simulink model "IEEE14_case"  (R2024b)
settings: Solver=FixedStepAuto  StartTime=0  StopTime=2  FixedStep=1e-7  RelTol=1e-3
values from neighbouring files (symbols this model uses):
  GFL_15_Bva = 0.009    [IEEE14_parameters.m]
  GFL_15_C_bus_pu = 7.179419    [IEEE14_parameters.m]
  GFL_15_f0 = 60    [IEEE14_parameters.m]
  GFL_15_I_id = 691.26967    [IEEE14_parameters.m]
  GFL_15_I_iq = 691.26967    [IEEE14_parameters.m]
  GFL_15_I_od = 45.2207    [IEEE14_parameters.m]
  GFL_15_I_oq = 45.2207    [IEEE14_parameters.m]
  GFL_15_I_pll = 0.78    [IEEE14_parameters.m]
  GFL_15_Kdi = 0.09    [IEEE14_parameters.m]
  GFL_15_Kdo = 0.9    [IEEE14_parameters.m]
  GFL_15_Kqi = 0.09    [IEEE14_parameters.m]
  GFL_15_Kqo = 0.9    [IEEE14_parameters.m]
  GFL_15_Lg_pu = 0.631447    [IEEE14_parameters.m]
  GFL_15_mode = 1    [IEEE14_parameters.m]
  GFL_15_P_id = 3.7166    [IEEE14_parameters.m]
  GFL_15_P_iq = 3.7166    [IEEE14_parameters.m]
  GFL_15_P_od = 0.4798    [IEEE14_parameters.m]
  GFL_15_P_oq = 0.4798    [IEEE14_parameters.m]
  GFL_15_P_pll = 290.42    [IEEE14_parameters.m]
  GFL_15_Qe_ref = 0.2    [IEEE14_parameters.m]
  GFL_15_Rg_pu = 0.024016    [IEEE14_parameters.m]
  GFL_15_Sbase = 1.000000e+4    (= 10000)    [IEEE14_parameters.m]
  GFL_15_Tdi = 0.01    [IEEE14_parameters.m]
  GFL_15_Tdo = 0.2    [IEEE14_parameters.m]
  GFL_15_Tqi = 0.01    [IEEE14_parameters.m]
  GFL_15_Tqo = 0.2    [IEEE14_parameters.m]
  GFL_15_Vbase = 380    [IEEE14_parameters.m]
  GFL_15_Vdc_ref = 1.011475    [IEEE14_parameters.m]
  GFL_15_Vdcbase = 700    [IEEE14_parameters.m]
  GFL_15_vq_ref = 0    [IEEE14_parameters.m]
  GFL_16_Bva = 0.002    [IEEE14_parameters.m]
  GFL_16_C_bus_pu = 7.179419    [IEEE14_parameters.m]
  GFL_16_f0 = 60    [IEEE14_parameters.m]
  GFL_16_I_id = 691.26967    [IEEE14_parameters.m]
  GFL_16_I_iq = 691.26967    [IEEE14_parameters.m]
  GFL_16_I_od = 45.2207    [IEEE14_parameters.m]
  GFL_16_I_oq = 45.2207    [IEEE14_parameters.m]
  GFL_16_I_pll = 0.78    [IEEE14_parameters.m]
  GFL_16_Kdi = 0.05    [IEEE14_parameters.m]
  GFL_16_Kdo = 0.5    [IEEE14_parameters.m]
  GFL_16_Kqi = 0.05    [IEEE14_parameters.m]
  GFL_16_Kqo = 0.5    [IEEE14_parameters.m]
  GFL_16_Lg_pu = 0.631447    [IEEE14_parameters.m]
  GFL_16_mode = 1    [IEEE14_parameters.m]
  GFL_16_P_id = 3.7166    [IEEE14_parameters.m]
  GFL_16_P_iq = 3.7166    [IEEE14_parameters.m]
  GFL_16_P_od = 0.4798    [IEEE14_parameters.m]
  GFL_16_P_oq = 0.4798    [IEEE14_parameters.m]
  GFL_16_P_pll = 290.42    [IEEE14_parameters.m]
  GFL_16_Qe_ref = 0.2    [IEEE14_parameters.m]
  GFL_16_Rg_pu = 0.024016    [IEEE14_parameters.m]
  GFL_16_Sbase = 1.000000e+4    (= 10000)    [IEEE14_parameters.m]
  GFL_16_Tdi = 0.01    [IEEE14_parameters.m]
  GFL_16_Tdo = 0.2    [IEEE14_parameters.m]
  GFL_16_Tqi = 0.01    [IEEE14_parameters.m]
  GFL_16_Tqo = 0.2    [IEEE14_parameters.m]
  GFL_16_Vbase = 380    [IEEE14_parameters.m]
  GFL_16_Vdc_ref = 1.01144    [IEEE14_parameters.m]
  GFL_16_Vdcbase = 700    [IEEE14_parameters.m]
  GFL_16_vq_ref = 0    [IEEE14_parameters.m]
  GFL_17_Bva = 0.002    [IEEE14_parameters.m]
  GFL_17_C_bus_pu = 7.179419    [IEEE14_parameters.m]
  GFL_17_f0 = 60    [IEEE14_parameters.m]
  GFL_17_I_id = 691.26967    [IEEE14_parameters.m]
  GFL_17_I_iq = 691.26967    [IEEE14_parameters.m]
  GFL_17_I_od = 45.2207    [IEEE14_parameters.m]
  GFL_17_I_oq = 45.2207    [IEEE14_parameters.m]
  GFL_17_I_pll = 0.78    [IEEE14_parameters.m]
  GFL_17_Kdi = 0.05    [IEEE14_parameters.m]
  GFL_17_Kdo = 0.5    [IEEE14_parameters.m]
  GFL_17_Kqi = 0.05    [IEEE14_parameters.m]
  GFL_17_Kqo = 0.5    [IEEE14_parameters.m]
  GFL_17_Lg_pu = 0.631447    [IEEE14_parameters.m]
  GFL_17_mode = 1    [IEEE14_parameters.m]
  GFL_17_P_id = 3.7166    [IEEE14_parameters.m]
  GFL_17_P_iq = 3.7166    [IEEE14_parameters.m]
  GFL_17_P_od = 0.4798    [IEEE14_parameters.m]
  GFL_17_P_oq = 0.4798    [IEEE14_parameters.m]
  GFL_17_P_pll = 290.42    [IEEE14_parameters.m]
  GFL_17_Qe_ref = 0.2    [IEEE14_parameters.m]
  GFL_17_Rg_pu = 0.024016    [IEEE14_parameters.m]
  GFL_17_Sbase = 1.000000e+4    (= 10000)    [IEEE14_parameters.m]
  GFL_17_Tdi = 0.01    [IEEE14_parameters.m]
  GFL_17_Tdo = 0.2    [IEEE14_parameters.m]
  GFL_17_Tqi = 0.01    [IEEE14_parameters.m]
  GFL_17_Tqo = 0.2    [IEEE14_parameters.m]
  GFL_17_Vbase = 380    [IEEE14_parameters.m]
  GFL_17_Vdc_ref = 1.011632    [IEEE14_parameters.m]
  GFL_17_Vdcbase = 700    [IEEE14_parameters.m]
  GFL_17_vq_ref = 0    [IEEE14_parameters.m]
  GFL_18_Bva = 0.002    [IEEE14_parameters.m]
  GFL_18_C_bus_pu = 7.179419    [IEEE14_parameters.m]
  GFL_18_f0 = 60    [IEEE14_parameters.m]
  GFL_18_I_id = 691.26967    [IEEE14_parameters.m]
  GFL_18_I_iq = 691.26967    [IEEE14_parameters.m]
  GFL_18_I_od = 45.2207    [IEEE14_parameters.m]
  GFL_18_I_oq = 45.2207    [IEEE14_parameters.m]
  GFL_18_I_pll = 0.78    [IEEE14_parameters.m]
  GFL_18_Kdi = 0.05    [IEEE14_parameters.m]
  GFL_18_Kdo = 0.5    [IEEE14_parameters.m]
  GFL_18_Kqi = 0.05    [IEEE14_parameters.m]
  GFL_18_Kqo = 0.5    [IEEE14_parameters.m]
  GFL_18_Lg_pu = 0.631447    [IEEE14_parameters.m]
  GFL_18_mode = 1    [IEEE14_parameters.m]
  GFL_18_P_id = 3.7166    [IEEE14_parameters.m]
  GFL_18_P_iq = 3.7166    [IEEE14_parameters.m]
  GFL_18_P_od = 0.4798    [IEEE14_parameters.m]
  GFL_18_P_oq = 0.4798    [IEEE14_parameters.m]
  GFL_18_P_pll = 290.42    [IEEE14_parameters.m]
  GFL_18_Qe_ref = 0.2    [IEEE14_parameters.m]
  GFL_18_Rg_pu = 0.024016    [IEEE14_parameters.m]
  GFL_18_Sbase = 1.000000e+4    (= 10000)    [IEEE14_parameters.m]
  GFL_18_Tdi = 0.01    [IEEE14_parameters.m]
  GFL_18_Tdo = 0.2    [IEEE14_parameters.m]
  GFL_18_Tqi = 0.01    [IEEE14_parameters.m]
  GFL_18_Tqo = 0.2    [IEEE14_parameters.m]
  GFL_18_Vbase = 380    [IEEE14_parameters.m]
  GFL_18_Vdc_ref = 1.011572    [IEEE14_parameters.m]
  GFL_18_Vdcbase = 700    [IEEE14_parameters.m]
  GFL_18_vq_ref = 0    [IEEE14_parameters.m]
  ... (+180 more)
(part 24 of 25)

== system IEEE14_case/SG_D_8/d_psi_fd_SG_D_8_block ==
  note: d_psi_fd_SG_D_8 in case14gfl
      | $-\frac{\psi _{\mathrm{fd},\mathrm{SG},D,8}-E_{\mathrm{fd},\mathrm{SG},D,8}+\left(x_{d}-x_{\mathrm{dd}}\right)\,\left(\frac{\frac{\psi _{\mathrm{1d},\mathrm{SG},D,8}\,\left(x_{\mathrm{dd}}-x_{\mathrm{ddd}}\right)}{x_{\mathrm{dd}}-x_{l}}-\psi _{d,\mathrm{SG},D,8}+\frac{\psi _{\mathrm{fd},\mathrm{SG},D,8}\,\left(x_{\mathrm{ddd}}-x_{l}\right)}{x_{\mathrm{dd}}-x_{l}}}{x_{\mathrm{ddd}}}-\frac{\left(x_{\mathrm{dd}}-x_{\mathrm{ddd}}\right)\,\left(\psi _{\mathrm{1d},\mathrm{SG},D,8}-\psi _{\mathrm{fd},\mathrm{SG},D,8}+\frac{\left(x_{\mathrm{dd}}-x_{l}\right)\,\left(\frac{\psi _{\mathrm{1d},\mathrm{SG},D,8}\,\left(x_{\mathrm{dd}}-x_{\mathrm{ddd}}\right)}{x_{\mathrm{dd}}-x_{l}}-\psi _{d,\mathrm{SG},D,8}+\frac{\psi _{\mathrm{fd},\mathrm{SG},D,8}\,\left(x_{\mathrm{ddd}}-x_{l}\right)}{x_{\mathrm{dd}}-x_{l}}\right)}{x_{\mathrm{ddd}}}\right)}{{\left(x_{\mathrm{dd}}-x_{l}\right)}^2}\right)}{T_{\mathrm{dd}}}$
      | Automatically generated on 2025-10-09 21:33:59 .
  State_E_fd_SG_D_8_e02cf : Inport
  State_psi_fd_SG_D_8_39b4d : Inport  Port=2
  State_psi_1d_SG_D_8_31c78 : Inport  Port=3
  State_psi_fd_SG_D_8_1b7c8 : Inport  Port=4
  State_psi_1d_SG_D_8_9e1bf : Inport  Port=5
  State_psi_d_SG_D_8_43284 : Inport  Port=6
  State_psi_fd_SG_D_8_ed057 : Inport  Port=7
  State_psi_1d_SG_D_8_5095e : Inport  Port=8
  State_psi_d_SG_D_8_8f483 : Inport  Port=9
  State_psi_fd_SG_D_8_f6f0f : Inport  Port=10
  Add_26f22 : Sum
  Add_5b217 : Sum
  Constant_-1_26542 : Constant  Value=-1
  Constant_-1_3797d : Constant  Value=-1
  Constant_-1_dec03 : Constant  Value=-1
  Constant_2.0_3ed6d : Constant  Value=2.0
  Constant_T_dd_0dbbc : Constant  Value=T_dd
  Constant_x_d_6bf3f : Constant  Value=x_d
  Constant_x_dd_0b8c2 : Constant  Value=x_dd
  Constant_x_dd_34914 : Constant  Value=x_dd
  Constant_x_dd_4f598 : Constant  Value=x_dd
  Constant_x_dd_7273b : Constant  Value=x_dd
  Constant_x_dd_8c3c1 : Constant  Value=x_dd
  Constant_x_dd_8e3a0 : Constant  Value=x_dd
  Constant_x_dd_a5c14 : Constant  Value=x_dd
  Constant_x_dd_b5d33 : Constant  Value=x_dd
  Constant_x_dd_bee28 : Constant  Value=x_dd
  Constant_x_dd_fd05b : Constant  Value=x_dd
  Constant_x_ddd_1d51c : Constant  Value=x_ddd
  Constant_x_ddd_45ab1 : Constant  Value=x_ddd
  Constant_x_ddd_4919d : Constant  Value=x_ddd
  Constant_x_ddd_7d5f3 : Constant  Value=x_ddd
  Constant_x_ddd_7fc36 : Constant  Value=x_ddd
  Constant_x_ddd_a00fc : Constant  Value=x_ddd
  Constant_x_ddd_af341 : Constant  Value=x_ddd
  Constant_x_l_0f4c1 : Constant  Value=x_l
  Constant_x_l_47282 : Constant  Value=x_l
  Constant_x_l_89ab3 : Constant  Value=x_l
  Constant_x_l_986fb : Constant  Value=x_l
  Constant_x_l_b3eb1 : Constant  Value=x_l
  Constant_x_l_b6760 : Constant  Value=x_l
  Constant_x_l_bcff8 : Constant  Value=x_l
  Constant_x_l_f5a13 : Constant  Value=x_l
  Divide_25bb4 : Product  Inputs=*/
  Divide_26f02 : Product  Inputs=*/
  Divide_49211 : Product  Inputs=*/
  Divide_521f5 : Product  Inputs=*/
  Divide_6930e : Product  Inputs=*/
  Divide_99e34 : Product  Inputs=*/
  Divide_a134a : Product  Inputs=*/
  Divide_d8446 : Product  Inputs=*/
  Power_ac428 : Math  Operator=pow
  Product_1dea7 : Product
  Product_1f0ee : Product
  Product_2c675 : Product
  Product_48aea : Product
  Product_704ec : Product
  Product_729c8 : Product
  Product_8251c : Product
  Product_a93fa : Product
  Product_b88eb : Product
  Product_c49e1 : Product
  Subtract_129ea : Sum  Inputs=+-
  Subtract_1642a : Sum  Inputs=+-
  Subtract_19a77 : Sum  Inputs=+-
  Subtract_2e5e4 : Sum  Inputs=+-
  Subtract_348eb : Sum  Inputs=+-
  Subtract_439c9 : Sum  Inputs=+-
  Subtract_5895d : Sum  Inputs=+-
  Subtract_6887b : Sum  Inputs=+-
  Subtract_777f5 : Sum  Inputs=+-
  Subtract_7f03a : Sum  Inputs=+-
  Subtract_9a066 : Sum  Inputs=+-
  Subtract_a91ef : Sum  Inputs=+-
  Subtract_b472e : Sum  Inputs=+-
  Subtract_ba576 : Sum  Inputs=+-
  Subtract_c05d3 : Sum  Inputs=+-
  Subtract_dfbb9 : Sum  Inputs=+-
  Subtract_e7edc : Sum  Inputs=+-
  Subtract_f439d : Sum  Inputs=+-
  Subtract_fe665 : Sum  Inputs=+-
  Blockout_d_psi_fd_SG_D_8_d8ca3 : Outport
  wires:
  Constant_x_l_0f4c1/1 -> Subtract_fe665/2
  Constant_-1_dec03/1 -> Product_a93fa/1
  Constant_x_dd_34914/1 -> Subtract_fe665/1
  State_psi_1d_SG_D_8_9e1bf/1 -> Product_a93fa/2
  Constant_x_dd_a5c14/1 -> Subtract_439c9/1
  Constant_x_ddd_4919d/1 -> Subtract_ba576/2
  Constant_x_dd_4f598/1 -> Subtract_ba576/1
  Constant_x_ddd_45ab1/1 -> Subtract_439c9/2
  Constant_x_ddd_af341/1 -> Divide_a134a/2
  Product_a93fa/1 -> Product_c49e1/1
  Subtract_439c9/1 -> Product_c49e1/2
  Constant_-1_3797d/1 -> Product_b88eb/1
  Constant_x_ddd_1d51c/1 -> Subtract_6887b/1
  Constant_x_l_89ab3/1 -> Subtract_6887b/2
  Constant_x_l_b6760/1 -> Subtract_777f5/2
  Product_c49e1/1 -> Divide_6930e/1
  Subtract_fe665/1 -> Divide_6930e/2
  State_psi_fd_SG_D_8_ed057/1 -> Product_1dea7/1
  Subtract_6887b/1 -> Product_1dea7/2
  Constant_x_dd_0b8c2/1 -> Subtract_19a77/1
  Constant_x_dd_bee28/1 -> Subtract_f439d/1
  Constant_-1_26542/1 -> Product_8251c/1
  Constant_x_l_b3eb1/1 -> Subtract_f439d/2
  Divide_6930e/1 -> Add_5b217/1
  State_psi_d_SG_D_8_43284/1 -> Add_5b217/2
  Product_2c675/1 -> Divide_521f5/1
  Product_1dea7/1 -> Divide_99e34/1
  Subtract_f439d/1 -> Divide_99e34/2
  Constant_x_l_bcff8/1 -> Subtract_19a77/2
  Add_5b217/1 -> Subtract_9a066/1
  Divide_99e34/1 -> Subtract_9a066/2
  Subtract_348eb/1 -> Subtract_e7edc/1
  State_psi_1d_SG_D_8_5095e/1 -> Product_8251c/2
  Subtract_ba576/1 -> Product_b88eb/2
  Constant_x_dd_8c3c1/1 -> Subtract_a91ef/1
  Subtract_129ea/1 -> Power_ac428/1
  Constant_x_ddd_7fc36/1 -> Subtract_a91ef/2
  Product_704ec/1 -> Divide_26f02/1
  Subtract_19a77/1 -> Product_2c675/1
  Constant_x_l_986fb/1 -> Subtract_5895d/2
  Product_48aea/1 -> Subtract_7f03a/2
  Subtract_9a066/1 -> Product_2c675/2
  Product_8251c/1 -> Product_704ec/1
  State_psi_1d_SG_D_8_31c78/1 -> Subtract_348eb/1
  Subtract_a91ef/1 -> Product_704ec/2
  Constant_x_dd_b5d33/1 -> Subtract_1642a/1
  Constant_x_l_f5a13/1 -> Subtract_1642a/2
  Subtract_5895d/1 -> Product_729c8/2
  Constant_x_ddd_7d5f3/1 -> Subtract_5895d/1
  State_psi_fd_SG_D_8_1b7c8/1 -> Subtract_348eb/2
  Subtract_1642a/1 -> Divide_26f02/2
  Constant_x_ddd_a00fc/1 -> Divide_521f5/2
  Product_729c8/1 -> Divide_49211/1
  State_psi_fd_SG_D_8_f6f0f/1 -> Product_729c8/1
  Subtract_777f5/1 -> Divide_49211/2
  Constant_x_dd_8e3a0/1 -> Subtract_777f5/1
  Divide_521f5/1 -> Subtract_e7edc/2
  Constant_x_dd_fd05b/1 -> Subtract_129ea/1
  Divide_49211/1 -> Subtract_c05d3/2
  Constant_2.0_3ed6d/1 -> Power_ac428/2
  Constant_x_l_47282/1 -> Subtract_129ea/2
  Divide_26f02/1 -> Add_26f22/1
  State_psi_d_SG_D_8_8f483/1 -> Add_26f22/2
  Product_b88eb/1 -> Product_1f0ee/1
  Add_26f22/1 -> Subtract_c05d3/1
  Subtract_e7edc/1 -> Product_1f0ee/2
  Product_1f0ee/1 -> Divide_d8446/1
  Power_ac428/1 -> Divide_d8446/2
  Subtract_c05d3/1 -> Divide_a134a/1
  Constant_x_d_6bf3f/1 -> Subtract_b472e/1
  Constant_x_dd_7273b/1 -> Subtract_b472e/2
  Divide_d8446/1 -> Subtract_dfbb9/1
  Divide_a134a/1 -> Subtract_dfbb9/2
  State_E_fd_SG_D_8_e02cf/1 -> Subtract_2e5e4/1
  State_psi_fd_SG_D_8_39b4d/1 -> Subtract_2e5e4/2
  Subtract_b472e/1 -> Product_48aea/1
  Subtract_dfbb9/1 -> Product_48aea/2
  Subtract_2e5e4/1 -> Subtract_7f03a/1
  Subtract_7f03a/1 -> Divide_25bb4/1
  Constant_T_dd_0dbbc/1 -> Divide_25bb4/2
  Divide_25bb4/1 -> Blockout_d_psi_fd_SG_D_8_d8ca3/1

== system IEEE14_case/SG_D_8/d_psi_gq_SG_D_8_block ==
  note: d_psi_gq_SG_D_8 in case14gfl
      | $-\frac{\psi _{\mathrm{gq},\mathrm{SG},D,8}+\left(x_{q}-x_{\mathrm{qd}}\right)\,\left(\frac{\psi _{q,\mathrm{SG},D,8}+\frac{\psi _{\mathrm{gq},\mathrm{SG},D,8}\,\left(x_{l}-x_{\mathrm{qdd}}\right)}{x_{l}-x_{\mathrm{qd}}}+\frac{\psi _{\mathrm{kq},\mathrm{SG},D,8}\,\left(x_{\mathrm{qd}}-x_{\mathrm{qdd}}\right)}{x_{l}-x_{\mathrm{qd}}}}{x_{\mathrm{qdd}}}+\frac{\left(x_{\mathrm{qd}}-x_{\mathrm{qdd}}\right)\,\left(\psi _{\mathrm{gq},\mathrm{SG},D,8}+\psi _{\mathrm{kq},\mathrm{SG},D,8}+\frac{\left(x_{l}-x_{\mathrm{qd}}\right)\,\left(\psi _{q,\mathrm{SG},D,8}+\frac{\psi _{\mathrm{gq},\mathrm{SG},D,8}\,\left(x_{l}-x_{\mathrm{qdd}}\right)}{x_{l}-x_{\mathrm{qd}}}+\frac{\psi _{\mathrm{kq},\mathrm{SG},D,8}\,\left(x_{\mathrm{qd}}-x_{\mathrm{qdd}}\right)}{x_{l}-x_{\mathrm{qd}}}\right)}{x_{\mathrm{qdd}}}\right)}{{\left(x_{l}-x_{\mathrm{qd}}\right)}^2}\right)}{T_{\mathrm{qd}}}$
      | Automatically generated on 2025-10-09 21:34:07 .
  State_psi_gq_SG_D_8_21c0a : Inport
  State_psi_gq_SG_D_8_953e4 : Inport  Port=2
  State_psi_kq_SG_D_8_6a8ed : Inport  Port=3
  State_psi_gq_SG_D_8_d7d68 : Inport  Port=4
  State_psi_kq_SG_D_8_1ecc5 : Inport  Port=5
  State_psi_q_SG_D_8_5d8c1 : Inport  Port=6
  State_psi_gq_SG_D_8_869cf : Inport  Port=7
  State_psi_kq_SG_D_8_7be32 : Inport  Port=8
  State_psi_q_SG_D_8_ecb47 : Inport  Port=9
  Add_07730 : Sum
  Add_1ca26 : Sum
  Add_40510 : Sum
  Add_42d04 : Sum
  Add_4fd95 : Sum
  Add_60192 : Sum
  Add_9d762 : Sum
  Add_9d8b6 : Sum
  Add_a59c4 : Sum
  Add_b029c : Sum
  Add_b5da7 : Sum
  Add_ff199 : Sum
  Constant_-1_00251 : Constant  Value=-1
  Constant_-1_09ee5 : Constant  Value=-1
  Constant_-1_2d718 : Constant  Value=-1
  Constant_-1_48847 : Constant  Value=-1
  Constant_-1_4f652 : Constant  Value=-1
  Constant_-1_753a3 : Constant  Value=-1
  Constant_-1_a1e37 : Constant  Value=-1
  Constant_-1_a5330 : Constant  Value=-1
  Constant_-1_b6ee6 : Constant  Value=-1
  Constant_-1_e0751 : Constant  Value=-1
  Constant_2.0_4854f : Constant  Value=2.0
  Constant_T_qd_ffd75 : Constant  Value=T_qd
  Constant_x_l_0bfe3 : Constant  Value=x_l
  Constant_x_l_1dd7f : Constant  Value=x_l
  Constant_x_l_3d847 : Constant  Value=x_l
  Constant_x_l_3d87b : Constant  Value=x_l
  Constant_x_l_6a2c3 : Constant  Value=x_l
  Constant_x_l_95e58 : Constant  Value=x_l
  Constant_x_l_ab144 : Constant  Value=x_l
  Constant_x_l_d5b73 : Constant  Value=x_l
  Constant_x_q_6e1a0 : Constant  Value=x_q
  Constant_x_qd_14af0 : Constant  Value=x_qd
  Constant_x_qd_27253 : Constant  Value=x_qd
  Constant_x_qd_37a04 : Constant  Value=x_qd
  Constant_x_qd_5c3c1 : Constant  Value=x_qd
  Constant_x_qd_6a317 : Constant  Value=x_qd
  Constant_x_qd_6a685 : Constant  Value=x_qd
  Constant_x_qd_9bae0 : Constant  Value=x_qd
  Constant_x_qd_b0b28 : Constant  Value=x_qd
  Constant_x_qd_c841e : Constant  Value=x_qd
  Constant_x_qd_f6025 : Constant  Value=x_qd
  Constant_x_qdd_026b8 : Constant  Value=x_qdd
  Constant_x_qdd_08be3 : Constant  Value=x_qdd
  Constant_x_qdd_1ecb2 : Constant  Value=x_qdd
  Constant_x_qdd_3fa39 : Constant  Value=x_qdd
  Constant_x_qdd_57c15 : Constant  Value=x_qdd
  Constant_x_qdd_89854 : Constant  Value=x_qdd
  Constant_x_qdd_be84b : Constant  Value=x_qdd
  Divide_0acb9 : Product  Inputs=*/
  Divide_487d7 : Product  Inputs=*/
  Divide_50180 : Product  Inputs=*/
  Divide_6ce65 : Product  Inputs=*/
  Divide_9bf5f : Product  Inputs=*/
  Divide_adc13 : Product  Inputs=*/
  Divide_c3deb : Product  Inputs=*/
  Divide_f2596 : Product  Inputs=*/
  Power_740e1 : Math  Operator=pow
  Product_04446 : Product
  Product_08077 : Product
  Product_1852e : Product
  Product_3a9cc : Product
  Product_3fc6d : Product
  Product_450c9 : Product
  Product_6d480 : Product
  Product_7a0ba : Product
  Product_98db6 : Product
  Product_a784b : Product
  Product_a8122 : Product
  Product_c9044 : Product
  Product_e5b1b : Product
  Product_ed7d0 : Product
  Product_f1f97 : Product
  Product_f61b5 : Product
  Product_f8355 : Product
  Subtract_098c6 : Sum  Inputs=+-
  Subtract_44fb6 : Sum  Inputs=+-
  Subtract_4ed76 : Sum  Inputs=+-
  Subtract_603a0 : Sum  Inputs=+-
  Subtract_69945 : Sum  Inputs=+-
  Subtract_6e6a4 : Sum  Inputs=+-
  Subtract_8129e : Sum  Inputs=+-
  Subtract_901f5 : Sum  Inputs=+-
  Blockout_d_psi_gq_SG_D_8_03a58 : Outport
  wires:
  Constant_-1_a5330/1 -> Product_ed7d0/1
  Constant_x_l_d5b73/1 -> Product_ed7d0/2
  State_psi_kq_SG_D_8_1ecc5/1 -> Product_98db6/1
  Constant_x_l_6a2c3/1 -> Product_f1f97/2
  Product_ed7d0/1 -> Add_a59c4/1
  Subtract_4ed76/1 -> Product_98db6/2
  Constant_x_qdd_57c15/1 -> Add_a59c4/2
  Constant_-1_09ee5/1 -> Product_f1f97/1
  Divide_0acb9/1 -> Blockout_d_psi_gq_SG_D_8_03a58/1
  Constant_x_qd_9bae0/1 -> Subtract_4ed76/1
  Add_a59c4/1 -> Product_3a9cc/2
  Constant_x_qdd_be84b/1 -> Subtract_4ed76/2
  Constant_-1_48847/1 -> Product_450c9/1
  Constant_x_qdd_026b8/1 -> Subtract_69945/2
  Subtract_098c6/1 -> Add_07730/1
  Constant_x_l_0bfe3/1 -> Product_450c9/2
  State_psi_gq_SG_D_8_d7d68/1 -> Product_3a9cc/1
  Product_f1f97/1 -> Add_60192/1
  Constant_x_qd_b0b28/1 -> Add_1ca26/2
  Constant_x_qd_c841e/1 -> Add_60192/2
  Product_450c9/1 -> Add_40510/1
  Divide_adc13/1 -> Subtract_098c6/1
  Constant_x_qd_6a317/1 -> Add_40510/2
  Product_3a9cc/1 -> Divide_adc13/1
  Add_60192/1 -> Divide_adc13/2
  Product_98db6/1 -> Divide_6ce65/1
  State_psi_q_SG_D_8_5d8c1/1 -> Add_07730/2
  Add_40510/1 -> Divide_6ce65/2
  Constant_x_l_3d87b/1 -> Product_08077/2
  Product_1852e/1 -> Add_42d04/1
  Constant_-1_00251/1 -> Product_c9044/1
  Constant_x_l_3d847/1 -> Product_c9044/2
  Divide_6ce65/1 -> Subtract_098c6/2
  Constant_x_qd_37a04/1 -> Add_9d8b6/2
  Constant_-1_a1e37/1 -> Product_1852e/1
  Subtract_603a0/1 -> Product_a784b/2
  Product_08077/1 -> Add_9d8b6/1
  Constant_x_l_95e58/1 -> Product_1852e/2
  Product_c9044/1 -> Add_1ca26/1
  Constant_-1_2d718/1 -> Product_08077/1
  Constant_x_qdd_08be3/1 -> Add_42d04/2
  Constant_-1_4f652/1 -> Product_3fc6d/1
  Subtract_69945/1 -> Product_e5b1b/2
  Product_f61b5/1 -> Divide_487d7/1
  Constant_x_q_6e1a0/1 -> Subtract_6e6a4/1
  Constant_x_l_ab144/1 -> Product_3fc6d/2
  Constant_x_qd_27253/1 -> Subtract_8129e/1
  Divide_9bf5f/1 -> Subtract_44fb6/2
  Add_4fd95/1 -> Divide_487d7/2
  Constant_x_qdd_3fa39/1 -> Subtract_8129e/2
  Add_1ca26/1 -> Product_f8355/1
  Add_42d04/1 -> Product_f61b5/2
  Constant_x_qdd_89854/1 -> Divide_c3deb/2
  Add_07730/1 -> Product_f8355/2
  State_psi_gq_SG_D_8_869cf/1 -> Product_f61b5/1
  Product_3fc6d/1 -> Add_4fd95/1
  Product_f8355/1 -> Divide_9bf5f/1
  Constant_x_qd_6a685/1 -> Subtract_69945/1
  Constant_x_qd_5c3c1/1 -> Add_4fd95/2
  State_psi_kq_SG_D_8_7be32/1 -> Product_7a0ba/1
  Constant_x_l_1dd7f/1 -> Product_6d480/2
  Subtract_8129e/1 -> Product_7a0ba/2
  State_psi_gq_SG_D_8_953e4/1 -> Add_b5da7/1
  State_psi_kq_SG_D_8_6a8ed/1 -> Add_b5da7/2
  Constant_x_qdd_1ecb2/1 -> Divide_9bf5f/2
  Constant_-1_e0751/1 -> Product_6d480/1
  Product_7a0ba/1 -> Divide_50180/1
  Product_e5b1b/1 -> Product_a8122/1
  Add_9d8b6/1 -> Divide_50180/2
  Constant_-1_b6ee6/1 -> Product_e5b1b/1
  Add_b5da7/1 -> Subtract_44fb6/1
  Product_6d480/1 -> Add_b029c/1
  Constant_x_qd_f6025/1 -> Add_b029c/2
  Divide_487d7/1 -> Subtract_901f5/1
  Divide_50180/1 -> Subtract_901f5/2
  Subtract_44fb6/1 -> Product_a8122/2
  Add_b029c/1 -> Power_740e1/1
  Constant_2.0_4854f/1 -> Power_740e1/2
  Subtract_901f5/1 -> Add_ff199/1
  State_psi_q_SG_D_8_ecb47/1 -> Add_ff199/2
  Product_a8122/1 -> Divide_f2596/1
  Power_740e1/1 -> Divide_f2596/2
  Add_ff199/1 -> Divide_c3deb/1
  Constant_x_qd_14af0/1 -> Subtract_6e6a4/2
  Divide_f2596/1 -> Subtract_603a0/1
  Divide_c3deb/1 -> Subtract_603a0/2
  Constant_-1_753a3/1 -> Product_04446/1
  State_psi_gq_SG_D_8_21c0a/1 -> Product_04446/2
  Subtract_6e6a4/1 -> Product_a784b/1
  Product_04446/1 -> Add_9d762/1
  Product_a784b/1 -> Add_9d762/2
  Add_9d762/1 -> Divide_0acb9/1
  Constant_T_qd_ffd75/1 -> Divide_0acb9/2

== system IEEE14_case/SG_D_8/d_psi_kq_SG_D_8_block ==
  note: d_psi_kq_SG_D_8 in case14gfl
      | $-\frac{\psi _{\mathrm{gq},\mathrm{SG},D,8}+\psi _{\mathrm{kq},\mathrm{SG},D,8}+\frac{\left(x_{l}-x_{\mathrm{qd}}\right)\,\left(\psi _{q,\mathrm{SG},D,8}+\frac{\psi _{\mathrm{gq},\mathrm{SG},D,8}\,\left(x_{l}-x_{\mathrm{qdd}}\right)}{x_{l}-x_{\mathrm{qd}}}+\frac{\psi _{\mathrm{kq},\mathrm{SG},D,8}\,\left(x_{\mathrm{qd}}-x_{\mathrm{qdd}}\right)}{x_{l}-x_{\mathrm{qd}}}\right)}{x_{\mathrm{qdd}}}}{T_{\mathrm{qdd}}}$
      | Automatically generated on 2025-10-09 21:34:10 .
  State_psi_gq_SG_D_8_46c2d : Inport
  State_psi_kq_SG_D_8_36a8a : Inport  Port=2
  State_psi_gq_SG_D_8_4cdf1 : Inport  Port=3
  State_psi_kq_SG_D_8_90e06 : Inport  Port=4
  State_psi_q_SG_D_8_6f170 : Inport  Port=5
  Add_28f8c : Sum
  Add_401a4 : Sum
  Add_806d9 : Sum
  Add_adae5 : Sum
  Add_ecaa8 : Sum
  Add_fbc6b : Sum
  Constant_-1_31262 : Constant  Value=-1
  Constant_-1_75045 : Constant  Value=-1
  Constant_-1_bb471 : Constant  Value=-1
  Constant_-1_d3138 : Constant  Value=-1
  Constant_-1_e202b : Constant  Value=-1
  Constant_T_qdd_cfb7e : Constant  Value=T_qdd
  Constant_x_l_2431d : Constant  Value=x_l
  Constant_x_l_381c4 : Constant  Value=x_l
  Constant_x_l_6de6a : Constant  Value=x_l
  Constant_x_l_e798a : Constant  Value=x_l
  Constant_x_qd_156f6 : Constant  Value=x_qd
  Constant_x_qd_51847 : Constant  Value=x_qd
  Constant_x_qd_5c479 : Constant  Value=x_qd
  Constant_x_qd_bc859 : Constant  Value=x_qd
  Constant_x_qdd_356d2 : Constant  Value=x_qdd
  Constant_x_qdd_5aff9 : Constant  Value=x_qdd
  Constant_x_qdd_93a4d : Constant  Value=x_qdd
  Divide_1cc31 : Product  Inputs=*/
  Divide_71367 : Product  Inputs=*/
  Divide_8a730 : Product  Inputs=*/
  Divide_db037 : Product  Inputs=*/
  Product_0104e : Product
  Product_187c8 : Product
  Product_6fb44 : Product
  Product_72a72 : Product
  Product_81b50 : Product
  Product_94e03 : Product
  Product_95910 : Product
  Product_d587f : Product
  Subtract_a1c9b : Sum  Inputs=+-
  Subtract_b1d1f : Sum  Inputs=+-
  Subtract_ea2f8 : Sum  Inputs=+-
  Blockout_d_psi_kq_SG_D_8_f1e70 : Outport
  wires:
  Constant_-1_75045/1 -> Product_0104e/1
  Constant_-1_31262/1 -> Product_187c8/1
  Constant_x_l_381c4/1 -> Product_0104e/2
  Constant_x_qdd_356d2/1 -> Add_adae5/2
  Constant_x_l_6de6a/1 -> Product_187c8/2
  Constant_-1_e202b/1 -> Product_6fb44/1
  Product_187c8/1 -> Add_adae5/1
  Constant_x_qd_5c479/1 -> Subtract_ea2f8/1
  Constant_x_qdd_93a4d/1 -> Subtract_ea2f8/2
  Constant_x_l_e798a/1 -> Product_6fb44/2
  State_psi_gq_SG_D_8_4cdf1/1 -> Product_81b50/1
  Add_adae5/1 -> Product_81b50/2
  Product_0104e/1 -> Add_ecaa8/1
  Subtract_b1d1f/1 -> Add_fbc6b/1
  Constant_x_qd_156f6/1 -> Add_ecaa8/2
  State_psi_gq_SG_D_8_46c2d/1 -> Product_94e03/2
  Constant_x_l_2431d/1 -> Product_95910/2
  Product_81b50/1 -> Divide_71367/1
  State_psi_kq_SG_D_8_90e06/1 -> Product_72a72/1
  Subtract_ea2f8/1 -> Product_72a72/2
  Product_6fb44/1 -> Add_28f8c/1
  Divide_1cc31/1 -> Blockout_d_psi_kq_SG_D_8_f1e70/1
  Add_806d9/1 -> Product_d587f/1
  Constant_x_qd_bc859/1 -> Add_28f8c/2
  Add_ecaa8/1 -> Divide_71367/2
  Product_72a72/1 -> Divide_8a730/1
  Add_28f8c/1 -> Divide_8a730/2
  Constant_-1_d3138/1 -> Product_95910/1
  Divide_71367/1 -> Subtract_b1d1f/1
  Divide_8a730/1 -> Subtract_b1d1f/2
  Product_95910/1 -> Add_806d9/1
  Constant_x_qd_51847/1 -> Add_806d9/2
  State_psi_q_SG_D_8_6f170/1 -> Add_fbc6b/2
  Constant_-1_bb471/1 -> Product_94e03/1
  Add_fbc6b/1 -> Product_d587f/2
  Product_94e03/1 -> Subtract_a1c9b/1
  State_psi_kq_SG_D_8_36a8a/1 -> Subtract_a1c9b/2
  Product_d587f/1 -> Divide_db037/1
  Constant_x_qdd_5aff9/1 -> Divide_db037/2
  Subtract_a1c9b/1 -> Add_401a4/1
  Divide_db037/1 -> Add_401a4/2
  Add_401a4/1 -> Divide_1cc31/1
  Constant_T_qdd_cfb7e/1 -> Divide_1cc31/2

== system IEEE14_case/SG_D_8/d_psi_q_SG_D_8_block ==
  note: d_psi_q_SG_D_8 in case14gfl
      | $2\,\pi \,f_{0}\,\left(v_{d,\mathrm{SG},D,8}\,\cos\left(\theta _{\mathrm{SG},D,8}\right)+v_{q,\mathrm{SG},D,8}\,\sin\left(\theta _{\mathrm{SG},D,8}\right)-\frac{R_{a}\,\left(\psi _{q,\mathrm{SG},D,8}+\frac{\psi _{\mathrm{gq},\mathrm{SG},D,8}\,\left(x_{l}-x_{\mathrm{qdd}}\right)}{x_{l}-x_{\mathrm{qd}}}+\frac{\psi _{\mathrm{kq},\mathrm{SG},D,8}\,\left(x_{\mathrm{qd}}-x_{\mathrm{qdd}}\right)}{x_{l}-x_{\mathrm{qd}}}\right)}{x_{\mathrm{qdd}}}-\frac{\psi _{d,\mathrm{SG},D,8}\,w_{\mathrm{SG},D,8}}{2\,f_{0}\,\pi }\right)$
      | Automatically generated on 2025-10-09 21:33:55 .
  State_psi_gq_SG_D_8_a7fd3 : Inport
  State_psi_kq_SG_D_8_644c1 : Inport  Port=2
  State_psi_q_SG_D_8_e0430 : Inport  Port=3
  Input_v_d_SG_D_8_c09e8 : Inport  Port=4
  State_theta_SG_D_8_01782 : Inport  Port=5
  Input_v_q_SG_D_8_1ed15 : Inport  Port=6
  State_theta_SG_D_8_5a3fa : Inport  Port=7
  State_psi_d_SG_D_8_332cc : Inport  Port=8
  State_w_SG_D_8_716c2 : Inport  Port=9
  Add_30cbe : Sum
  Add_92e9c : Sum
  Add_955b2 : Sum
  Add_c26b3 : Sum
  Add_e58e6 : Sum
  Constant_-1_10d0a : Constant  Value=-1
  Constant_-1_6cfe9 : Constant  Value=-1
  Constant_-1_d3256 : Constant  Value=-1
  Constant_-2.0_555a1 : Constant  Value=-2.0
  Constant_2.0_728c1 : Constant  Value=2.0
  Constant_R_a_3e55b : Constant  Value=R_a
  Constant_f0_3f887 : Constant  Value=f0
  Constant_f0_b8e22 : Constant  Value=f0
  Constant_pi_6da32 : Constant  Value=pi
  Constant_pi_8f741 : Constant  Value=pi
  Constant_x_l_6c7eb : Constant  Value=x_l
  Constant_x_l_7d638 : Constant  Value=x_l
  Constant_x_l_e1b36 : Constant  Value=x_l
  Constant_x_qd_21134 : Constant  Value=x_qd
  Constant_x_qd_51a46 : Constant  Value=x_qd
  Constant_x_qd_e51c6 : Constant  Value=x_qd
  Constant_x_qdd_391b0 : Constant  Value=x_qdd
  Constant_x_qdd_3c426 : Constant  Value=x_qdd
  Constant_x_qdd_6e24d : Constant  Value=x_qdd
  Divide_23286 : Product  Inputs=*/
  Divide_8a514 : Product  Inputs=*/
  Divide_94bdd : Product  Inputs=*/
  Divide_a85fb : Product  Inputs=*/
  MathFunc_cos_23bfe : Trigonometry  Operator=cos
  MathFunc_sin_571b0 : Trigonometry
  Product_11c7a : Product
  Product_1b665 : Product
  Product_1e979 : Product
  Product_33f02 : Product
  Product_37ec4 : Product
  Product_3d04a : Product
  Product_8176b : Product
  Product_90596 : Product
  Product_ba7fd : Product
  Product_c0862 : Product
  Product_d3987 : Product
  Product_d4bb6 : Product
  Product_eda59 : Product
  Product_fe6f4 : Product
  Subtract_0e403 : Sum  Inputs=+-
  Subtract_3104a : Sum  Inputs=+-
  Subtract_4cf1c : Sum  Inputs=+-
  Subtract_b2507 : Sum  Inputs=+-
  Blockout_d_psi_q_SG_D_8_90d0e : Outport
  wires:
  MathFunc_cos_23bfe/1 -> Product_ba7fd/2
  State_theta_SG_D_8_01782/1 -> MathFunc_cos_23bfe/1
  Constant_x_l_6c7eb/1 -> Product_3d04a/2
  Constant_-1_6cfe9/1 -> Product_c0862/1
  Constant_x_l_e1b36/1 -> Product_c0862/2
  Divide_8a514/1 -> Add_92e9c/2
  Constant_x_qdd_6e24d/1 -> Subtract_3104a/2
  Product_37ec4/1 -> Product_1b665/1
  Product_c0862/1 -> Add_c26b3/1
  State_w_SG_D_8_716c2/1 -> Product_fe6f4/2
  Constant_x_qd_21134/1 -> Subtract_3104a/1
  Constant_x_qdd_391b0/1 -> Add_c26b3/2
  Add_30cbe/1 -> Product_33f02/2
  Constant_-1_d3256/1 -> Product_3d04a/1
  Constant_-1_10d0a/1 -> Product_1e979/1
  Product_d3987/1 -> Subtract_0e403/2
  Input_v_q_SG_D_8_1ed15/1 -> Product_d3987/1
  Constant_x_l_7d638/1 -> Product_1e979/2
  Divide_23286/1 -> Subtract_b2507/1
  State_psi_gq_SG_D_8_a7fd3/1 -> Product_eda59/1
  Add_c26b3/1 -> Product_eda59/2
  Product_3d04a/1 -> Add_955b2/1
  Constant_x_qd_51a46/1 -> Add_955b2/2
  State_psi_kq_SG_D_8_644c1/1 -> Product_d4bb6/1
  Subtract_3104a/1 -> Product_d4bb6/2
  Product_1e979/1 -> Add_e58e6/1
  MathFunc_sin_571b0/1 -> Product_d3987/2
  Constant_x_qd_e51c6/1 -> Add_e58e6/2
  Product_eda59/1 -> Divide_a85fb/1
  Add_955b2/1 -> Divide_a85fb/2
  State_psi_q_SG_D_8_e0430/1 -> Add_30cbe/2
  Product_d4bb6/1 -> Divide_94bdd/1
  Add_e58e6/1 -> Divide_94bdd/2
  Divide_a85fb/1 -> Subtract_4cf1c/1
  Divide_94bdd/1 -> Subtract_4cf1c/2
  Product_11c7a/1 -> Product_90596/1
  Subtract_4cf1c/1 -> Add_30cbe/1
  Subtract_b2507/1 -> Subtract_0e403/1
  Constant_R_a_3e55b/1 -> Product_33f02/1
  Constant_f0_3f887/1 -> Product_37ec4/2
  Constant_pi_6da32/1 -> Product_11c7a/2
  Product_33f02/1 -> Divide_23286/1
  Constant_x_qdd_3c426/1 -> Divide_23286/2
  Input_v_d_SG_D_8_c09e8/1 -> Product_ba7fd/1
  State_theta_SG_D_8_5a3fa/1 -> MathFunc_sin_571b0/1
  Constant_2.0_728c1/1 -> Product_11c7a/1
  Product_ba7fd/1 -> Subtract_b2507/2
  State_psi_d_SG_D_8_332cc/1 -> Product_fe6f4/1
  Subtract_0e403/1 -> Add_92e9c/1
  Constant_f0_b8e22/1 -> Product_90596/2
  Constant_-2.0_555a1/1 -> Product_8176b/1
  Constant_pi_8f741/1 -> Product_8176b/2
  Product_fe6f4/1 -> Divide_8a514/1
  Product_90596/1 -> Divide_8a514/2
  Product_8176b/1 -> Product_37ec4/1
  Add_92e9c/1 -> Product_1b665/2
  Product_1b665/1 -> Blockout_d_psi_q_SG_D_8_90d0e/1

== system IEEE14_case/SG_D_8/d_theta_SG_D_8_block ==
  note: d_theta_SG_D_8 in case14gfl
      | $w_{\mathrm{SG},D,8}-2\,\pi \,f_{0}$
      | Automatically generated on 2025-10-09 21:34:15 .
  State_w_SG_D_8_7874c : Inport
  Add_d0260 : Sum
  Constant_-2.0_deb9f : Constant  Value=-2.0
  Constant_f0_b0d24 : Constant  Value=f0
  Constant_pi_b9868 : Constant  Value=pi
  Product_39795 : Product
  Product_59a41 : Product
  Blockout_d_theta_SG_D_8_7fdd6 : Outport
  wires:
  Constant_-2.0_deb9f/1 -> Product_59a41/1
  Constant_pi_b9868/1 -> Product_59a41/2
  State_w_SG_D_8_7874c/1 -> Add_d0260/2
  Product_39795/1 -> Add_d0260/1
  Product_59a41/1 -> Product_39795/1
  Add_d0260/1 -> Blockout_d_theta_SG_D_8_7fdd6/1
  Constant_f0_b0d24/1 -> Product_39795/2

== system IEEE14_case/SG_D_8/d_w_SG_D_8_block ==
  note: d_w_SG_D_8 in case14gfl
      | $\frac{2\,\pi \,T_{m,\mathrm{SG},D,8}\,f_{0}-D\,\left(w_{\mathrm{SG},D,8}-2\,\pi \,f_{0}\right)+2\,\pi \,f_{0}\,\left(\frac{\psi _{d,\mathrm{SG},D,8}\,\left(\psi _{q,\mathrm{SG},D,8}+\frac{\psi _{\mathrm{gq},\mathrm{SG},D,8}\,\left(x_{l}-x_{\mathrm{qdd}}\right)}{x_{l}-x_{\mathrm{qd}}}+\frac{\psi _{\mathrm{kq},\mathrm{SG},D,8}\,\left(x_{\mathrm{qd}}-x_{\mathrm{qdd}}\right)}{x_{l}-x_{\mathrm{qd}}}\right)}{x_{\mathrm{qdd}}}+\frac{\psi _{q,\mathrm{SG},D,8}\,\left(\frac{\psi _{\mathrm{1d},\mathrm{SG},D,8}\,\left(x_{\mathrm{dd}}-x_{\mathrm{ddd}}\right)}{x_{\mathrm{dd}}-x_{l}}-\psi _{d,\mathrm{SG},D,8}+\frac{\psi _{\mathrm{fd},\mathrm{SG},D,8}\,\left(x_{\mathrm{ddd}}-x_{l}\right)}{x_{\mathrm{dd}}-x_{l}}\right)}{x_{\mathrm{ddd}}}\right)}{2\,H}$
      | Automatically generated on 2025-10-09 21:34:14 .
  State_w_SG_D_8_a443d : Inport
  State_T_m_SG_D_8_49ad0 : Inport  Port=2
  State_psi_d_SG_D_8_19a89 : Inport  Port=3
  State_psi_gq_SG_D_8_6cde6 : Inport  Port=4
  State_psi_kq_SG_D_8_f145c : Inport  Port=5
  State_psi_q_SG_D_8_202ce : Inport  Port=6
  State_psi_q_SG_D_8_9c5c1 : Inport  Port=7
  State_psi_1d_SG_D_8_25d54 : Inport  Port=8
  State_psi_d_SG_D_8_5f3fa : Inport  Port=9
  State_psi_fd_SG_D_8_93d32 : Inport  Port=10
  Add_0e486 : Sum
  Add_0e7e0 : Sum
  Add_2fd2d : Sum
  Add_8c40b : Sum
  Add_b9e10 : Sum
  Add_c9612 : Sum
  Add_e05e7 : Sum
  Add_e942d : Sum
  Constant_-1_0b6cf : Constant  Value=-1
  Constant_-1_15f4d : Constant  Value=-1
  Constant_-1_43a89 : Constant  Value=-1
  Constant_-1_5cb2b : Constant  Value=-1
  Constant_-1_76a35 : Constant  Value=-1
  Constant_-1_ca941 : Constant  Value=-1
  Constant_-2.0_f45ce : Constant  Value=-2.0
  Constant_2.0_257e3 : Constant  Value=2.0
  Constant_2.0_57c00 : Constant  Value=2.0
  Constant_2.0_73003 : Constant  Value=2.0
  Constant_D_5b923 : Constant  Value=D
  Constant_H_5fea1 : Constant  Value=H
  Constant_f0_2940c : Constant  Value=f0
  Constant_f0_8fa51 : Constant  Value=f0
  Constant_f0_e5de1 : Constant  Value=f0
  Constant_pi_296fa : Constant  Value=pi
  Constant_pi_c7cff : Constant  Value=pi
  Constant_pi_d02a9 : Constant  Value=pi
  Constant_x_dd_07e83 : Constant  Value=x_dd
  Constant_x_dd_25175 : Constant  Value=x_dd
  Constant_x_dd_65500 : Constant  Value=x_dd
  Constant_x_ddd_1ac2e : Constant  Value=x_ddd
  Constant_x_ddd_be832 : Constant  Value=x_ddd
  Constant_x_ddd_cb1c4 : Constant  Value=x_ddd
  Constant_x_l_6fe30 : Constant  Value=x_l
  Constant_x_l_b4d55 : Constant  Value=x_l
  Constant_x_l_d7f9b : Constant  Value=x_l
  Constant_x_l_e15fb : Constant  Value=x_l
  Constant_x_l_e4ddd : Constant  Value=x_l
  Constant_x_l_f3a8c : Constant  Value=x_l
  Constant_x_qd_13138 : Constant  Value=x_qd
  Constant_x_qd_6ad60 : Constant  Value=x_qd
  Constant_x_qd_7c449 : Constant  Value=x_qd
  Constant_x_qdd_0e982 : Constant  Value=x_qdd
  Constant_x_qdd_2016f : Constant  Value=x_qdd
  Constant_x_qdd_8e033 : Constant  Value=x_qdd
  Divide_51a2a : Product  Inputs=*/
  Divide_52151 : Product  Inputs=*/
  Divide_7448f : Product  Inputs=*/
  Divide_8fd75 : Product  Inputs=*/
  Divide_a9ca7 : Product  Inputs=*/
  Divide_c9042 : Product  Inputs=*/
  Divide_e328d : Product  Inputs=*/
  Product_0658f : Product
  Product_08cb0 : Product
  Product_1016f : Product
  Product_1d9c1 : Product
  Product_2b235 : Product
  Product_2da38 : Product
  Product_45b77 : Product
  Product_69d63 : Product
  Product_6b04b : Product
  Product_7b338 : Product
  Product_854fd : Product
  Product_b6a71 : Product
  Product_b74aa : Product
  Product_b8e58 : Product
  Product_ce9e9 : Product
  Product_e026c : Product
  Product_e1002 : Product
  Product_e6160 : Product
  Product_f3d28 : Product
  Product_f9c11 : Product
  Product_f9e5f : Product
  Product_fb406 : Product
  Subtract_2d695 : Sum  Inputs=+-
  Subtract_59904 : Sum  Inputs=+-
  Subtract_72ab7 : Sum  Inputs=+-
  Subtract_a6a1e : Sum  Inputs=+-
  Subtract_b36b8 : Sum  Inputs=+-
  Subtract_b5695 : Sum  Inputs=+-
  Subtract_c3889 : Sum  Inputs=+-
  Subtract_d1c6d : Sum  Inputs=+-
  Blockout_d_w_SG_D_8_91fe0 : Outport
  wires:
  Constant_2.0_73003/1 -> Product_f9e5f/1
  Constant_pi_296fa/1 -> Product_b74aa/2
  Constant_x_l_b4d55/1 -> Product_e6160/2
  State_w_SG_D_8_a443d/1 -> Add_e05e7/2
  Constant_-1_0b6cf/1 -> Product_69d63/1
  Product_69d63/1 -> Add_c9612/1
  Constant_x_l_e15fb/1 -> Product_69d63/2
  Subtract_c3889/1 -> Product_1d9c1/2
  Constant_x_qd_6ad60/1 -> Subtract_c3889/1
  Constant_x_qdd_2016f/1 -> Add_c9612/2
  Constant_x_l_e4ddd/1 -> Subtract_b5695/2
  Product_e6160/1 -> Add_0e486/1
  Constant_-1_76a35/1 -> Product_e6160/1
  Constant_x_qdd_8e033/1 -> Subtract_c3889/2
  Constant_-1_43a89/1 -> Product_ce9e9/1
  State_psi_d_SG_D_8_5f3fa/1 -> Add_0e7e0/2
  Product_ce9e9/1 -> Add_b9e10/1
  Subtract_b36b8/1 -> Divide_52151/2
  Constant_x_l_d7f9b/1 -> Product_ce9e9/2
  Constant_-1_15f4d/1 -> Product_2b235/1
  State_psi_1d_SG_D_8_25d54/1 -> Product_2b235/2
  State_psi_q_SG_D_8_202ce/1 -> Add_e942d/2
  Constant_x_dd_25175/1 -> Subtract_72ab7/1
  Constant_x_ddd_1ac2e/1 -> Subtract_72ab7/2
  Product_b8e58/1 -> Divide_a9ca7/1
  State_psi_gq_SG_D_8_6cde6/1 -> Product_b8e58/1
  Add_c9612/1 -> Product_b8e58/2
  Product_2b235/1 -> Product_2da38/1
  Constant_x_qd_13138/1 -> Add_0e486/2
  Product_1d9c1/1 -> Divide_51a2a/1
  State_psi_kq_SG_D_8_f145c/1 -> Product_1d9c1/1
  Constant_x_dd_07e83/1 -> Subtract_b36b8/1
  Constant_x_qd_7c449/1 -> Add_b9e10/2
  Subtract_72ab7/1 -> Product_2da38/2
  Add_b9e10/1 -> Divide_51a2a/2
  Constant_x_l_6fe30/1 -> Subtract_b36b8/2
  Subtract_59904/1 -> Product_f3d28/2
  Divide_c9042/1 -> Blockout_d_w_SG_D_8_91fe0/1
  Constant_x_ddd_cb1c4/1 -> Subtract_59904/1
  Add_e942d/1 -> Product_fb406/2
  Constant_x_l_f3a8c/1 -> Subtract_59904/2
  Add_0e486/1 -> Divide_a9ca7/2
  Product_2da38/1 -> Divide_52151/1
  Constant_2.0_257e3/1 -> Product_1016f/1
  Product_f3d28/1 -> Divide_8fd75/1
  State_psi_fd_SG_D_8_93d32/1 -> Product_f3d28/1
  Constant_D_5b923/1 -> Product_854fd/2
  State_psi_d_SG_D_8_19a89/1 -> Product_e1002/2
  Subtract_b5695/1 -> Divide_8fd75/2
  Constant_x_dd_65500/1 -> Subtract_b5695/1
  Constant_pi_c7cff/1 -> Product_1016f/2
  Divide_a9ca7/1 -> Subtract_2d695/1
  Divide_51a2a/1 -> Subtract_2d695/2
  Divide_52151/1 -> Add_0e7e0/1
  Constant_-2.0_f45ce/1 -> Product_b74aa/1
  Product_e1002/1 -> Product_fb406/1
  Constant_-1_ca941/1 -> Product_e1002/1
  Subtract_2d695/1 -> Add_e942d/1
  Add_0e7e0/1 -> Subtract_d1c6d/1
  Divide_8fd75/1 -> Subtract_d1c6d/2
  Constant_-1_5cb2b/1 -> Product_854fd/1
  Product_fb406/1 -> Divide_7448f/1
  Product_b74aa/1 -> Product_45b77/1
  Constant_f0_8fa51/1 -> Product_45b77/2
  State_psi_q_SG_D_8_9c5c1/1 -> Product_e026c/1
  Subtract_d1c6d/1 -> Product_e026c/2
  Product_45b77/1 -> Add_e05e7/1
  Product_1016f/1 -> Product_7b338/1
  State_T_m_SG_D_8_49ad0/1 -> Product_7b338/2
  Constant_pi_d02a9/1 -> Product_f9e5f/2
  Constant_x_qdd_0e982/1 -> Divide_7448f/2
  Product_e026c/1 -> Divide_e328d/1
  Constant_x_ddd_be832/1 -> Divide_e328d/2
  Product_854fd/1 -> Product_08cb0/1
  Add_e05e7/1 -> Product_08cb0/2
  Product_7b338/1 -> Product_0658f/1
  Constant_f0_e5de1/1 -> Product_0658f/2
  Product_f9e5f/1 -> Product_6b04b/1
  Constant_f0_2940c/1 -> Product_6b04b/2
  Divide_7448f/1 -> Add_2fd2d/1
  Divide_e328d/1 -> Add_2fd2d/2
  Product_08cb0/1 -> Add_8c40b/1
  Product_0658f/1 -> Add_8c40b/2
  Product_6b04b/1 -> Product_b6a71/1
  Add_2fd2d/1 -> Product_b6a71/2
  Add_8c40b/1 -> Subtract_a6a1e/1
  Product_b6a71/1 -> Subtract_a6a1e/2
  Constant_2.0_57c00/1 -> Product_f9c11/1
  Constant_H_5fea1/1 -> Product_f9c11/2
  Subtract_a6a1e/1 -> Divide_c9042/1
  Product_f9c11/1 -> Divide_c9042/2

== system IEEE14_case/SG_D_8/i_d_SG_D_8_block ==
  note: i_d_SG_D_8 in case14gfl
      | $\frac{\sin\left(\theta _{\mathrm{SG},D,8}\right)\,\left(\frac{\psi _{\mathrm{1d},\mathrm{SG},D,8}\,\left(x_{\mathrm{dd}}-x_{\mathrm{ddd}}\right)}{x_{\mathrm{dd}}-x_{l}}-\psi _{d,\mathrm{SG},D,8}+\frac{\psi _{\mathrm{fd},\mathrm{SG},D,8}\,\left(x_{\mathrm{ddd}}-x_{l}\right)}{x_{\mathrm{dd}}-x_{l}}\right)}{x_{\mathrm{ddd}}}-\frac{\cos\left(\theta _{\mathrm{SG},D,8}\right)\,\left(\psi _{q,\mathrm{SG},D,8}+\frac{\psi _{\mathrm{gq},\mathrm{SG},D,8}\,\left(x_{l}-x_{\mathrm{qdd}}\right)}{x_{l}-x_{\mathrm{qd}}}+\frac{\psi _{\mathrm{kq},\mathrm{SG},D,8}\,\left(x_{\mathrm{qd}}-x_{\mathrm{qdd}}\right)}{x_{l}-x_{\mathrm{qd}}}\right)}{x_{\mathrm{qdd}}}$
      | Automatically generated on 2025-10-09 21:34:33 .
  State_psi_gq_SG_D_8_6ad23 : Inport
  State_psi_kq_SG_D_8_4cd34 : Inport  Port=2
  State_psi_q_SG_D_8_2ca29 : Inport  Port=3
  State_theta_SG_D_8_641e8 : Inport  Port=4
  State_psi_1d_SG_D_8_b3820 : Inport  Port=5
  State_psi_d_SG_D_8_f7e33 : Inport  Port=6
  State_psi_fd_SG_D_8_06311 : Inport  Port=7
  State_theta_SG_D_8_bcf58 : Inport  Port=8
  Add_2aeaa : Sum
  Add_4f32e : Sum
  Add_620a4 : Sum
  Add_79ad2 : Sum
  Add_ca698 : Sum
  Constant_-1_07394 : Constant  Value=-1
  Constant_-1_172d7 : Constant  Value=-1
  Constant_-1_63dfb : Constant  Value=-1
  Constant_-1_81eeb : Constant  Value=-1
  Constant_-1_a66d7 : Constant  Value=-1
  Constant_x_dd_01ebb : Constant  Value=x_dd
  Constant_x_dd_08d80 : Constant  Value=x_dd
  Constant_x_dd_f1948 : Constant  Value=x_dd
  Constant_x_ddd_6f589 : Constant  Value=x_ddd
  Constant_x_ddd_8370f : Constant  Value=x_ddd
  Constant_x_ddd_eb0fd : Constant  Value=x_ddd
  Constant_x_l_1a838 : Constant  Value=x_l
  Constant_x_l_49170 : Constant  Value=x_l
  Constant_x_l_70ddf : Constant  Value=x_l
  Constant_x_l_c499b : Constant  Value=x_l
  Constant_x_l_c7f83 : Constant  Value=x_l
  Constant_x_l_ee1cb : Constant  Value=x_l
  Constant_x_qd_1fe2a : Constant  Value=x_qd
  Constant_x_qd_6c938 : Constant  Value=x_qd
  Constant_x_qd_84ddc : Constant  Value=x_qd
  Constant_x_qdd_0423f : Constant  Value=x_qdd
  Constant_x_qdd_91bb8 : Constant  Value=x_qdd
  Constant_x_qdd_9738a : Constant  Value=x_qdd
  Divide_6412d : Product  Inputs=*/
  Divide_8ed95 : Product  Inputs=*/
  Divide_a2daa : Product  Inputs=*/
  Divide_aacd2 : Product  Inputs=*/
  Divide_ee12a : Product  Inputs=*/
  Divide_f8105 : Product  Inputs=*/
  MathFunc_cos_b838e : Trigonometry  Operator=cos
  MathFunc_sin_d00a2 : Trigonometry
  Product_26260 : Product
  Product_3488a : Product
  Product_469ef : Product
  Product_548ee : Product
  Product_57d20 : Product
  Product_61cd5 : Product
  Product_6a93a : Product
  Product_e0673 : Product
  Product_e7e6d : Product
  Product_e83a3 : Product
  Product_ed78a : Product
  Subtract_0991e : Sum  Inputs=+-
  Subtract_3811b : Sum  Inputs=+-
  Subtract_4d92d : Sum  Inputs=+-
  Subtract_6fb36 : Sum  Inputs=+-
  Subtract_7fdd0 : Sum  Inputs=+-
  Subtract_8747e : Sum  Inputs=+-
  Subtract_b22b8 : Sum  Inputs=+-
  Subtract_e0621 : Sum  Inputs=+-
  Blockout_i_d_SG_D_8_0f0f6 : Outport
  wires:
  Constant_x_qdd_9738a/1 -> Add_4f32e/2
  Subtract_b22b8/1 -> Blockout_i_d_SG_D_8_0f0f6/1
  Product_3488a/1 -> Product_26260/1
  Constant_-1_07394/1 -> Product_61cd5/1
  Product_61cd5/1 -> Add_4f32e/1
  Subtract_0991e/1 -> Divide_f8105/2
  Constant_x_dd_01ebb/1 -> Subtract_0991e/1
  Constant_x_l_1a838/1 -> Product_61cd5/2
  Constant_-1_81eeb/1 -> Product_ed78a/1
  Constant_x_qd_1fe2a/1 -> Subtract_6fb36/1
  Divide_8ed95/1 -> Add_79ad2/1
  Constant_x_l_ee1cb/1 -> Product_ed78a/2
  Constant_x_qdd_0423f/1 -> Subtract_6fb36/2
  Constant_-1_63dfb/1 -> Product_e0673/1
  Constant_-1_a66d7/1 -> Product_57d20/1
  Constant_x_l_49170/1 -> Product_e0673/2
  Add_620a4/1 -> Divide_6412d/2
  State_psi_gq_SG_D_8_6ad23/1 -> Product_469ef/1
  Constant_x_ddd_eb0fd/1 -> Divide_a2daa/2
  Add_4f32e/1 -> Product_469ef/2
  Product_ed78a/1 -> Add_2aeaa/1
  Product_e83a3/1 -> Divide_a2daa/1
  Constant_x_qd_84ddc/1 -> Add_2aeaa/2
  State_psi_kq_SG_D_8_4cd34/1 -> Product_548ee/1
  Product_469ef/1 -> Divide_aacd2/1
  Subtract_6fb36/1 -> Product_548ee/2
  Product_e0673/1 -> Add_620a4/1
  Constant_x_qd_6c938/1 -> Add_620a4/2
  Subtract_e0621/1 -> Add_ca698/1
  State_psi_1d_SG_D_8_b3820/1 -> Product_57d20/2
  Constant_x_dd_08d80/1 -> Subtract_7fdd0/1
  Constant_x_ddd_6f589/1 -> Subtract_7fdd0/2
  Divide_ee12a/1 -> Subtract_b22b8/1
  Constant_x_l_70ddf/1 -> Subtract_8747e/2
  Add_2aeaa/1 -> Divide_aacd2/2
  Constant_x_qdd_91bb8/1 -> Divide_ee12a/2
  Constant_-1_172d7/1 -> Product_3488a/1
  Product_548ee/1 -> Divide_6412d/1
  Product_57d20/1 -> Product_e7e6d/1
  Subtract_7fdd0/1 -> Product_e7e6d/2
  Constant_x_dd_f1948/1 -> Subtract_3811b/1
  Constant_x_l_c499b/1 -> Subtract_3811b/2
  Subtract_8747e/1 -> Product_6a93a/2
  Constant_x_ddd_8370f/1 -> Subtract_8747e/1
  Constant_x_l_c7f83/1 -> Subtract_0991e/2
  Divide_aacd2/1 -> Subtract_e0621/1
  Add_ca698/1 -> Product_3488a/2
  Divide_6412d/1 -> Subtract_e0621/2
  State_psi_q_SG_D_8_2ca29/1 -> Add_ca698/2
  Product_e7e6d/1 -> Divide_8ed95/1
  Subtract_3811b/1 -> Divide_8ed95/2
  Product_6a93a/1 -> Divide_f8105/1
  State_psi_fd_SG_D_8_06311/1 -> Product_6a93a/1
  State_psi_d_SG_D_8_f7e33/1 -> Add_79ad2/2
  MathFunc_cos_b838e/1 -> Product_26260/2
  State_theta_SG_D_8_641e8/1 -> MathFunc_cos_b838e/1
  Add_79ad2/1 -> Subtract_4d92d/1
  Divide_f8105/1 -> Subtract_4d92d/2
  MathFunc_sin_d00a2/1 -> Product_e83a3/2
  State_theta_SG_D_8_bcf58/1 -> MathFunc_sin_d00a2/1
  Subtract_4d92d/1 -> Product_e83a3/1
  Product_26260/1 -> Divide_ee12a/1
  Divide_a2daa/1 -> Subtract_b22b8/2
